simulink subsystem "PositionErrors"  (R2020a)
settings: Solver=VariableStepAuto  StartTime=0.0  StopTime=10.0  RelTol=1e-3
settings Model: Creator=charlie  LastModifiedBy=charlie

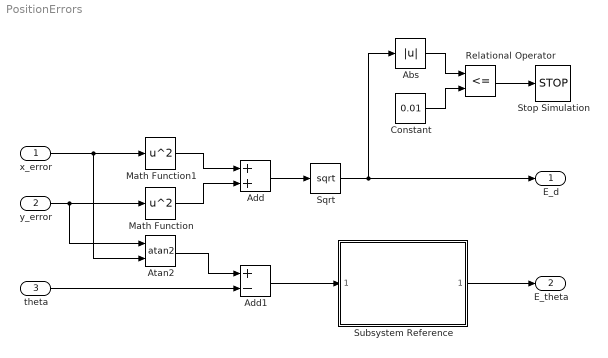
== system PositionErrors ==
  x_error : Inport
  y_error : Inport  Port=2
  theta : Inport  Port=3
  Abs : Abs
  Add : Sum
  Add1 : Sum  Inputs=+-
  Atan2 : Trigonometry  Operator=atan2
  Constant : Constant  Value=0.01
  Math Function : Math  Operator=square  SaturateOnIntegerOverflow=on
  Math Function1 : Math  Operator=square  SaturateOnIntegerOverflow=on
  Relational Operator : RelationalOperator  Operator=<=  OutDataTypeStr=boolean  RndMeth=Simplest
  Sqrt : Sqrt  SaturateOnIntegerOverflow=on
  Stop Simulation : Stop
  Subsystem Reference : Subsystem  ReferencedSubsystem=RangoTheta
  E_d : Outport
  E_theta : Outport  Port=2
  wires:
  Sqrt/1 -> Abs/1, E_d/1
  Math Function1/1 -> Add/1
  Relational Operator/1 -> Stop Simulation/1
  Subsystem Reference/1 -> E_theta/1
  Constant/1 -> Relational Operator/2
  Math Function/1 -> Add/2
  x_error/1 -> Atan2/2, Math Function1/1
  Add1/1 -> Subsystem Reference/1
  y_error/1 -> Atan2/1, Math Function/1
  Abs/1 -> Relational Operator/1
  Add/1 -> Sqrt/1
  theta/1 -> Add1/2
  Atan2/1 -> Add1/1
